simulink model "LQRR"  (R2015a)
settings: Solver=ode45  StartTime=0.0  StopTime=10.0  RelTol=1e-3
values from neighbouring files (symbols this model uses):
  A = [0,1,0;(mb*lb+mw*l)*g/(Ib+mw*(l^2)),-Cb/(Ib+mw*(l^2)),Cw/(Ib+mw*(l^2));-(mb*lb+mw*l)*g/(Ib+mw*(l^2)),Cb/(Ib+mw*(l^2)),-Cw*(Ib+Iw+mw*(l^2))/(Ib+mw*(l^2))/Iw]    [CubliFunction.m]
  B = [0;-Km/(Ib+mw*(l^2));Km*(Ib+Iw+mw*(l^2))/(Ib+mw*(l^2))/Iw]    [CubliFunction.m]
  C = eye(3)    [CubliFunction.m]
  D = zeros(3,1)    [CubliFunction.m]
  K1 = K(1,1)    [CubliFunction.m]
  K2 = K(1,2)    [CubliFunction.m]
  K3 = K(1,3)    [CubliFunction.m]
settings Model: Creator=Remy  LastModifiedBy=Remy

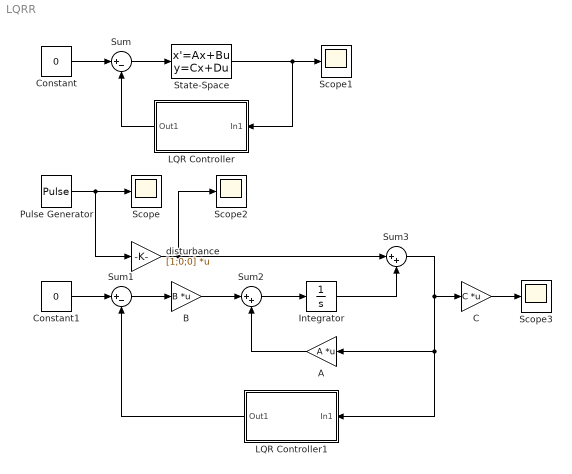
== system LQRR ==
  A : Gain  Gain=A  Multiplication=Matrix(K*u) (u vector)
  B : Gain  Gain=B  Multiplication=Matrix(K*u)
  C : Gain  Gain=C  Multiplication=Matrix(K*u)
  Constant : Constant  Value=0
  Constant1 : Constant  Value=0
  Integrator : Integrator
  LQR Controller : Subsystem  mask(LQR Controller){K1=K1, K2=K2, K3=K3}
  LQR Controller1 : Subsystem  mask(LQR Controller){K1=K1, K2=K2, K3=K3}
  Pulse Generator : DiscretePulseGenerator  PulseType=Time based  Amplitude=0.1  Period=10  PhaseDelay=1
  Scope{,1..3} (4 alike) : Scope
      Scope1 settings: ShowLegends=on
      Scope2 settings: ShowLegends=on  SaveName=ScopeData2
      Scope3 settings: ShowLegends=on  SaveName=ScopeData3
  State-Space : StateSpace  A=A  B=B  C=C  D=D  X0=[0.1;0;0]  ContinuousStateAttributes={'a', 'b', 'c'}
  Sum : Sum  Inputs=|+-
  Sum1 : Sum  Inputs=|+-
  Sum2 : Sum  Inputs=|++
  Sum3 : Sum  Inputs=|++
  disturbance : Gain  Gain=[1;0;0]  Multiplication=Matrix(K*u)
  wires:
  State-Space/1 -> Scope1/1, LQR Controller/1(In1)
  Sum/1 -> State-Space/1
  LQR Controller/1(Out1) -> Sum/2
  Constant/1 -> Sum/1
  Pulse Generator/1 -> Scope/1, disturbance/1
  disturbance/1 -> Scope2/1, Sum3/1
  Sum1/1 -> B/1
  LQR Controller1/1(Out1) -> Sum1/2
  Constant1/1 -> Sum1/1
  B/1 -> Sum2/1
  Sum2/1 -> Integrator/1
  C/1 -> Scope3/1
  A/1 -> Sum2/2
  Integrator/1 -> Sum3/2
  Sum3/1 -> LQR Controller1/1(In1), A/1, C/1

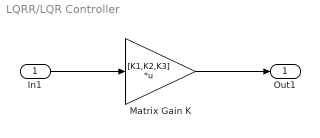
== system LQRR/LQR Controller ==
  In1 : Inport
  Matrix Gain K : Gain  Gain=[K1,K2,K3]  Multiplication=Matrix(K*u)
  Out1 : Outport
  wires:
  In1/1 -> Matrix Gain K/1
  Matrix Gain K/1 -> Out1/1

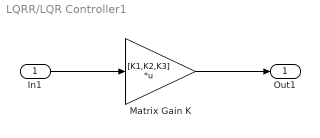
== system LQRR/LQR Controller1 ==
  In1 : Inport
  Matrix Gain K : Gain  Gain=[K1,K2,K3]  Multiplication=Matrix(K*u)
  Out1 : Outport
  wires:
  In1/1 -> Matrix Gain K/1
  Matrix Gain K/1 -> Out1/1
